simulink model "small_signal_box"  (R2024b)
settings: Solver=VariableStepAuto  StartTime=0.0  StopTime=Tobs  FixedStep=Ts  RelTol=1e-3
values from neighbouring files (symbols this model uses):
  P_finalvalue = 0.486    [main_scan_FD.m]    (also in main_ss_composite.m = 0.05)
  P_initialvalue = storage    (= 0.486)    [main_ss_composite.m]
  P_step = 0.05    [main_ss_composite.m]
  P_step_time = 1.5    [main_scan_FD.m]    (also in main_ss_composite.m = 10)
  Ts = delta_t    (= 1e-05)    [main_scan_FD.m]
  V_finalvalue = 0.99    [main_ss_composite.m]
  V_step_time = 100    [main_scan_FD.m]    (also in main_ss_composite.m = 10)
undefined symbols (not defined in the file or in its folder): C_dc, C_filt, I_charge, ig_d_s, ig_q_s, iL_d_s, iL_q_s, ki_inner_d_pu, ki_inner_q_pu, ki_outer_P_pu, ki_outer_V_pu, ki_pll, kp_inner_d_pu, kp_inner_q_pu, kp_outer_P_pu, kp_outer_V_pu, kp_pll, L, L_base, L_grid, L_vsc, omega_b, P_base, R_grid, R_vsc, t_charge, V_base, V_dc, vdc_mes, vpoc_d_s, vpoc_q_s, vvsc_d_s, vvsc_q_s
libraries: spsabctodq0Lib x8, spsControlledVoltageSourceLib x6, slpidlib x5, spsThreePhaseSeriesRLCBranchLib x3, spsControlledCurrentSourceLib x2, eeGeneralControl x2, spsdq0toabcLib x2, spsThreePhaseVIMeasurementLib x2, spsGroundLib x1, spsLeadLagFilterLib x1, spsParallelRLCBranchLib x1, cstblocks x1
settings Model: SimulationMode=accelerator  Creator=osro  LastModifiedBy=nicolae.darii
settings SolverCC: AlgebraicLoopSolver=TrustRegion
settings DataIOCC: SaveFinalState=on
settings DebuggingCC: UnconnectedInputMsg=warning  UnconnectedOutputMsg=warning  UnconnectedLineMsg=warning
settings ModelReferenceCC: EnableRefExpFcnMdlSchedulingChecks=on
settings RTWCC: GPUComputeCapability=3.5

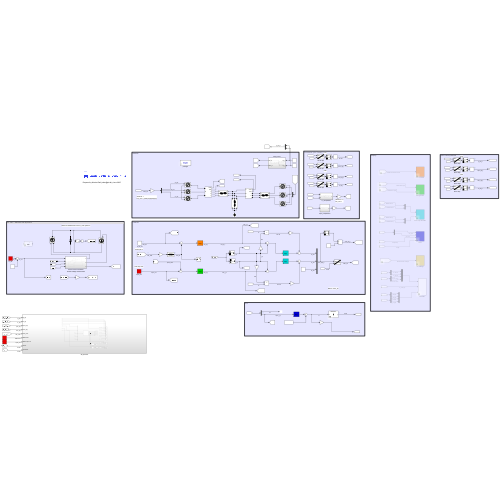
[thumbnail: Simulink's stored preview of the top-level diagram]
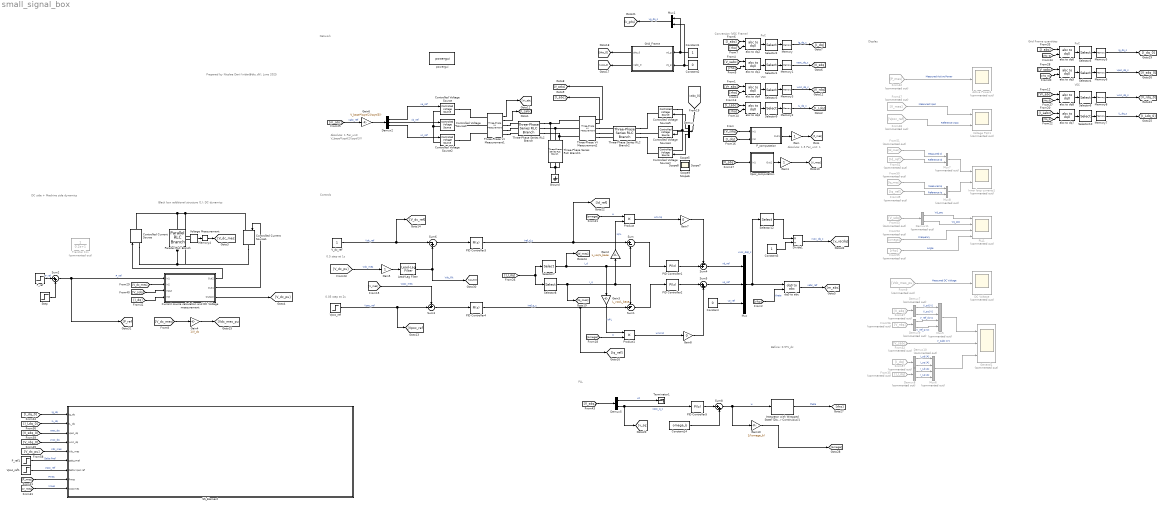
== system small_signal_box ==
  note: Before: 0.5*V_dc
  note: PLL
  note: 0.05 step at 2s
  note: 0.5 step at 1s
  note: Absolute: 1.5
      | Per_unit: 1
  note: Absolute: 1
      | Per_unit: V_base*(sqrt(2)/sqrt(3))
  note: Conversion (VSC Frame)
  note: Controls
  note: Network
  note: VSC
  note: PoC
  note: Prepared by Nicolae Darii (nidar@dtu.dk), June 2025
  note: DC side + Machine side dynamics
  note: Black box additional structure (1): DC dynamics
  note: Display
  note: VSC
  note: Grid Frame quantities
  note: PoC
  Active Power1 : Scope  Commented=on
  Constant : Constant  Value=0
  Constant1 : Constant
  Constant14 : Constant  Value=omega_b
  Constant2 : Constant  Value=0
  Constant3 : Constant
  Controlled Current Source : spsControlledCurrentSourceLib/Controlled Current Source  Initialize=on  Source_Type=AC  Amplitude=0  Phase=0  Frequency=0  Measurements=None
  Controlled Current Source1 : spsControlledCurrentSourceLib/Controlled Current Source  Initialize=on  Source_Type=AC  Amplitude=0  Phase=0  Frequency=0  Measurements=None
  Controlled Voltage Source{,1..5} (6 alike) : spsControlledVoltageSourceLib/Controlled Voltage Source  Initialize=on  Source_Type=AC  Amplitude=0  Phase=0  Frequency=0  Measurements=None
  Current source calculation and DC Voltage measurement : Subsystem
  DC Voltage : Scope  Commented=on
  Demux : Demux  Outputs=3
  Demux{7..11} (5 alike) : Demux  Commented=on  Outputs=2
  Demux2 : Demux  Outputs=3
  Demux5 : Demux  Outputs=2
  Divide1 : Product  Inputs=*/
  From32 : From  Commented=on  GotoTag=V_sabc
  From35 : From  Commented=on  GotoTag=I_Ldq
  From37 : From  Commented=on  GotoTag=V_sdq
  From42 : From  Commented=on  GotoTag=P_mes
  From47 : From  Commented=on  GotoTag=V_mes
  From48 : From  Commented=on  GotoTag=Vpoc_ref
  From49 : From  Commented=on  GotoTag=Iq_ref
  From50 : From  Commented=on  GotoTag=Iq_mes
  From51 : From  Commented=on  GotoTag=Id_mes
  From52 : From  Commented=on  GotoTag=Id_ref
  From53 : From  Commented=on  GotoTag=V_sdq
  From54 : From  Commented=on  GotoTag=omega
  From55 : From  Commented=on  GotoTag=rho
  From56 : From  Commented=on  GotoTag=V_rdq
  From57 : From  Commented=on  GotoTag=I_dq
  From9 : From  Commented=on  GotoTag=Vdc_mes_pu
  Gain : Gain
  Gain1 : Gain
  Gain10 : Gain  Gain=1/(omega_b)
  Gain2 : Gain  Gain=L_vsc/L_base
  Gain3 : Gain  Gain=L_vsc/L_base
  Gain4 : Gain  Gain=1/V_dc
  Gain5 : Gain
  Gain6 : Gain  Gain=V_base*(sqrt(2)/sqrt(3))
  Gain7 : Gain  Gain=0
  Gain8 : Gain  Gain=0
  General1 : Scope  Commented=on  NumInputPorts=3
  Grid_Frame : Subsystem
  Ground : spsGroundLib/Ground  LConnTagsString=a
  Inner loop currents1 : Scope  Commented=on  NumInputPorts=2
  Integrator with Wrapped State (Discrete or Continuous)1 : eeGeneralControl/Integrator with Wrapped State (Discrete or Continuous)  LabelModeActiveChoice=Discrete  WrappedStateUpperValue=2*pi  WrappedStateLowerValue=0  x0=0  Ts=-1
  Lead-Lag Filter : spsLeadLagFilterLib/Lead-Lag Filter  T1=T1  T2=T2  Vdc_Init=1  Ts=Ts
      settings: LibrarySourceBlock=|
      | sps_lib/Control/Filters/Lead-Lag
      | Filter
  Memory{,1..3,5..8} (8 alike) : Memory  InitialCondition=[0 0]  InheritSampleTime=on  LinearizeMemory=on  LinearizeAsDelay=on
  Memory4 : Memory
  Mux : Mux  Inputs=3
  Mux1 : Mux  Inputs=2
  Mux5 : Mux  Commented=on
  Mux6 : Mux  Commented=on
  Mux7 : Mux  Commented=on  Inputs=2
  Mux8 : Mux  Commented=on  Inputs=2
  PID Controller1 : slpidlib/PID Controller  Controller=PI  Form=Parallel  TimeDomain=Discrete-time  UseExternalTs=off  SampleTime=Ts  IntegratorMethod=Forward Euler  FilterMethod=Forward Euler  ControllerParametersSource=internal  P=kp_inner_d_pu  I=ki_inner_d_pu  UseKiTs=off  D=0  UseExternalDerivativeSource=off  N=100  UseFilter=on  TunerSelectOption=Transfer Function Based (PID Tuner App)  InitialConditionSource=internal  InitialConditionForIntegrator=0  InitialConditionForFilter=0  DifferentiatorICPrevScaledInput=0  ExternalReset=none  TrackingMode=off  Kt=1  LimitOutput=off  SatLimitsSource=internal  UpperSaturationLimit=inf  LowerSaturationLimit=-inf  LinearizeAsGain=on  AntiWindupMode=none  Kb=1  LimitIntegrator=off  UpperIntegratorSaturationLimit=inf  LowerIntegratorSaturationLimit=-inf  POutMin=[]  POutMax=[]  IOutMin=[]  IOutMax=[]  DOutMin=[]  DOutMax=[]  NOutMin=[]  NOutMax=[]  SumOutMin=[]  SumOutMax=[]  SaturationOutMin=[]  SaturationOutMax=[]  PParamMin=[]  PParamMax=[]  IParamMin=[]  IParamMax=[]  DParamMin=[]  DParamMax=[]  NParamMin=[]  NParamMax=[]  KbParamMin=[]  KbParamMax=[]  KtParamMin=[]  KtParamMax=[]  KbOutMin=[]  KbOutMax=[]  KtOutMin=[]  KtOutMax=[]  IntegratorOutMin=[]  IntegratorOutMax=[]  FilterOutMin=[]  FilterOutMax=[]  SumI1OutMin=[]  SumI1OutMax=[]  SumI2OutMin=[]  SumI2OutMax=[]  SumI3OutMin=[]  SumI3OutMax=[]  SumI4OutMin=[]  SumI4OutMax=[]  SumDOutMin=[]  SumDOutMax=[]  DifferentiatorOutMin=[]  DifferentiatorOutMax=[]  FilterDiffOutCoefMin=[]  FilterDiffOutCoefMax=[]  ReciprocalOutMin=[]  ReciprocalOutMax=[]  SumDenOutMin=[]  SumDenOutMax=[]  SumNumOutMin=[]  SumNumOutMax=[]  DivideOutMin=[]  DivideOutMax=[]  UdiffTsProdOutMin=[]  UdiffTsProdOutMax=[]  NTsProdOutMin=[]  NTsProdOutMax=[]  UintegralTsProdOutMin=[]  UintegralTsProdOutMax=[]  UngainTsProdOutMin=[]  UngainTsProdOutMax=[]  ClampingZeroOutDataTypeStr=Inherit: Inherit via back propagation  ClampingZeroOutMin=[]  ClampingZeroOutMax=[]  FilterDenConstantOutDataTypeStr=Inherit: Inherit via back propagation  FilterDenConstantOutMin=[]  FilterDenConstantOutMax=[]  PCopyOutDataTypeStr=Inherit: Inherit via back propagation  PCopyOutMin=[]  PCopyOutMax=[]  NCopyOutDataTypeStr=Inherit: Inherit via back propagation  NCopyOutMin=[]  NCopyOutMax=[]  IntegratorContinuousStateAttributes=''  IntegratorStateIdentifier="\"Cd\""  IntegratorStateMustResolveToSignalObject=off  IntegratorRTWStateStorageClass=Auto  FilterContinuousStateAttributes=''  FilterStateMustResolveToSignalObject=off  FilterRTWStateStorageClass=Auto  ParallelPVariant=InternalParameters  IdealPVariant=Disabled  IVariant=InternalParameters  DVariant=Disabled  IntegratorVariant=Discrete  SatVariant=Disabled  AWVariant=Passthrough  PCopyVariant=Disabled  TRVariant=Disabled  FdbkBlocksVariant=Forward  IdealPFdbkVariant=Disabled  SatFdbkVariant=Disabled  DerivativeFilterVariant=Disabled  NVariant=Disabled  NCopyVariant=Disabled_SignalSpec  FilterICVariant=Disabled  IntegratorICVariant=InternalICs  ExternalResetVariant=Disabled  TRSumVariant=Passthrough  SumFdbkVariant=Disabled  SumVariant=Sum_PI  TsampFilterVariant=InternalTs  TsampNgainVariant=Passthrough  TsampIntegralVariant=Disabled_SignalSpec  ExternalSaturationOutDataTypeStr=Inherit: Same as second input  DerivativeSourceVariant=Disabled  PreIntVariant=InternalPreInt
  PID Controller2 : slpidlib/PID Controller  Controller=PI  Form=Parallel  TimeDomain=Discrete-time  UseExternalTs=off  SampleTime=Ts  IntegratorMethod=Forward Euler  FilterMethod=Forward Euler  ControllerParametersSource=internal  P=kp_inner_q_pu  I=ki_inner_q_pu  UseKiTs=off  D=0  UseExternalDerivativeSource=off  N=100  UseFilter=on  TunerSelectOption=Transfer Function Based (PID Tuner App)  InitialConditionSource=internal  InitialConditionForIntegrator=0  InitialConditionForFilter=0  DifferentiatorICPrevScaledInput=0  ExternalReset=none  TrackingMode=off  Kt=1  LimitOutput=off  SatLimitsSource=internal  UpperSaturationLimit=inf  LowerSaturationLimit=-inf  LinearizeAsGain=on  AntiWindupMode=none  Kb=1  LimitIntegrator=off  UpperIntegratorSaturationLimit=inf  LowerIntegratorSaturationLimit=-inf  POutMin=[]  POutMax=[]  IOutMin=[]  IOutMax=[]  DOutMin=[]  DOutMax=[]  NOutMin=[]  NOutMax=[]  SumOutMin=[]  SumOutMax=[]  SaturationOutMin=[]  SaturationOutMax=[]  PParamMin=[]  PParamMax=[]  IParamMin=[]  IParamMax=[]  DParamMin=[]  DParamMax=[]  NParamMin=[]  NParamMax=[]  KbParamMin=[]  KbParamMax=[]  KtParamMin=[]  KtParamMax=[]  KbOutMin=[]  KbOutMax=[]  KtOutMin=[]  KtOutMax=[]  IntegratorOutMin=[]  IntegratorOutMax=[]  FilterOutMin=[]  FilterOutMax=[]  SumI1OutMin=[]  SumI1OutMax=[]  SumI2OutMin=[]  SumI2OutMax=[]  SumI3OutMin=[]  SumI3OutMax=[]  SumI4OutMin=[]  SumI4OutMax=[]  SumDOutMin=[]  SumDOutMax=[]  DifferentiatorOutMin=[]  DifferentiatorOutMax=[]  FilterDiffOutCoefMin=[]  FilterDiffOutCoefMax=[]  ReciprocalOutMin=[]  ReciprocalOutMax=[]  SumDenOutMin=[]  SumDenOutMax=[]  SumNumOutMin=[]  SumNumOutMax=[]  DivideOutMin=[]  DivideOutMax=[]  UdiffTsProdOutMin=[]  UdiffTsProdOutMax=[]  NTsProdOutMin=[]  NTsProdOutMax=[]  UintegralTsProdOutMin=[]  UintegralTsProdOutMax=[]  UngainTsProdOutMin=[]  UngainTsProdOutMax=[]  ClampingZeroOutDataTypeStr=Inherit: Inherit via back propagation  ClampingZeroOutMin=[]  ClampingZeroOutMax=[]  FilterDenConstantOutDataTypeStr=Inherit: Inherit via back propagation  FilterDenConstantOutMin=[]  FilterDenConstantOutMax=[]  PCopyOutDataTypeStr=Inherit: Inherit via back propagation  PCopyOutMin=[]  PCopyOutMax=[]  NCopyOutDataTypeStr=Inherit: Inherit via back propagation  NCopyOutMin=[]  NCopyOutMax=[]  IntegratorContinuousStateAttributes=''  IntegratorStateIdentifier="\"Cq\""  IntegratorStateMustResolveToSignalObject=off  IntegratorRTWStateStorageClass=Auto  FilterContinuousStateAttributes=''  FilterStateMustResolveToSignalObject=off  FilterRTWStateStorageClass=Auto  ParallelPVariant=InternalParameters  IdealPVariant=Disabled  IVariant=InternalParameters  DVariant=Disabled  IntegratorVariant=Discrete  SatVariant=Disabled  AWVariant=Passthrough  PCopyVariant=Disabled  TRVariant=Disabled  FdbkBlocksVariant=Forward  IdealPFdbkVariant=Disabled  SatFdbkVariant=Disabled  DerivativeFilterVariant=Disabled  NVariant=Disabled  NCopyVariant=Disabled_SignalSpec  FilterICVariant=Disabled  IntegratorICVariant=InternalICs  ExternalResetVariant=Disabled  TRSumVariant=Passthrough  SumFdbkVariant=Disabled  SumVariant=Sum_PI  TsampFilterVariant=InternalTs  TsampNgainVariant=Passthrough  TsampIntegralVariant=Disabled_SignalSpec  ExternalSaturationOutDataTypeStr=Inherit: Same as second input  DerivativeSourceVariant=Disabled  PreIntVariant=InternalPreInt
  PID Controller3 : slpidlib/PID Controller  Controller=PI  Form=Parallel  TimeDomain=Discrete-time  UseExternalTs=off  SampleTime=Ts  IntegratorMethod=Forward Euler  FilterMethod=Forward Euler  ControllerParametersSource=internal  P=kp_outer_P_pu  I=ki_outer_P_pu  UseKiTs=off  D=0  UseExternalDerivativeSource=off  N=100  UseFilter=on  TunerSelectOption=Transfer Function Based (PID Tuner App)  InitialConditionSource=internal  InitialConditionForIntegrator=0  InitialConditionForFilter=0  DifferentiatorICPrevScaledInput=0  ExternalReset=none  TrackingMode=off  Kt=1  LimitOutput=off  SatLimitsSource=internal  UpperSaturationLimit=inf  LowerSaturationLimit=-inf  LinearizeAsGain=on  AntiWindupMode=none  Kb=1  LimitIntegrator=off  UpperIntegratorSaturationLimit=inf  LowerIntegratorSaturationLimit=-inf  POutMin=[]  POutMax=[]  IOutMin=[]  IOutMax=[]  DOutMin=[]  DOutMax=[]  NOutMin=[]  NOutMax=[]  SumOutMin=[]  SumOutMax=[]  SaturationOutMin=[]  SaturationOutMax=[]  PParamMin=[]  PParamMax=[]  IParamMin=[]  IParamMax=[]  DParamMin=[]  DParamMax=[]  NParamMin=[]  NParamMax=[]  KbParamMin=[]  KbParamMax=[]  KtParamMin=[]  KtParamMax=[]  KbOutMin=[]  KbOutMax=[]  KtOutMin=[]  KtOutMax=[]  IntegratorOutMin=[]  IntegratorOutMax=[]  FilterOutMin=[]  FilterOutMax=[]  SumI1OutMin=[]  SumI1OutMax=[]  SumI2OutMin=[]  SumI2OutMax=[]  SumI3OutMin=[]  SumI3OutMax=[]  SumI4OutMin=[]  SumI4OutMax=[]  SumDOutMin=[]  SumDOutMax=[]  DifferentiatorOutMin=[]  DifferentiatorOutMax=[]  FilterDiffOutCoefMin=[]  FilterDiffOutCoefMax=[]  ReciprocalOutMin=[]  ReciprocalOutMax=[]  SumDenOutMin=[]  SumDenOutMax=[]  SumNumOutMin=[]  SumNumOutMax=[]  DivideOutMin=[]  DivideOutMax=[]  UdiffTsProdOutMin=[]  UdiffTsProdOutMax=[]  NTsProdOutMin=[]  NTsProdOutMax=[]  UintegralTsProdOutMin=[]  UintegralTsProdOutMax=[]  UngainTsProdOutMin=[]  UngainTsProdOutMax=[]  ClampingZeroOutDataTypeStr=Inherit: Inherit via back propagation  ClampingZeroOutMin=[]  ClampingZeroOutMax=[]  FilterDenConstantOutDataTypeStr=Inherit: Inherit via back propagation  FilterDenConstantOutMin=[]  FilterDenConstantOutMax=[]  PCopyOutDataTypeStr=Inherit: Inherit via back propagation  PCopyOutMin=[]  PCopyOutMax=[]  NCopyOutDataTypeStr=Inherit: Inherit via back propagation  NCopyOutMin=[]  NCopyOutMax=[]  IntegratorContinuousStateAttributes=''  IntegratorStateIdentifier="\"WP\""  IntegratorStateMustResolveToSignalObject=off  IntegratorRTWStateStorageClass=Auto  FilterContinuousStateAttributes=''  FilterStateMustResolveToSignalObject=off  FilterRTWStateStorageClass=Auto  ParallelPVariant=InternalParameters  IdealPVariant=Disabled  IVariant=InternalParameters  DVariant=Disabled  IntegratorVariant=Discrete  SatVariant=Disabled  AWVariant=Passthrough  PCopyVariant=Disabled  TRVariant=Disabled  FdbkBlocksVariant=Forward  IdealPFdbkVariant=Disabled  SatFdbkVariant=Disabled  DerivativeFilterVariant=Disabled  NVariant=Disabled  NCopyVariant=Disabled_SignalSpec  FilterICVariant=Disabled  IntegratorICVariant=InternalICs  ExternalResetVariant=Disabled  TRSumVariant=Passthrough  SumFdbkVariant=Disabled  SumVariant=Sum_PI  TsampFilterVariant=InternalTs  TsampNgainVariant=Passthrough  TsampIntegralVariant=Disabled_SignalSpec  ExternalSaturationOutDataTypeStr=Inherit: Same as second input  DerivativeSourceVariant=Disabled  PreIntVariant=InternalPreInt
  PID Controller4 : slpidlib/PID Controller  Controller=PI  Form=Parallel  TimeDomain=Discrete-time  UseExternalTs=off  SampleTime=Ts  IntegratorMethod=Forward Euler  FilterMethod=Forward Euler  ControllerParametersSource=internal  P=abs(kp_outer_V_pu)  I=abs(ki_outer_V_pu)  UseKiTs=off  D=0  UseExternalDerivativeSource=off  N=100  UseFilter=on  TunerSelectOption=Transfer Function Based (PID Tuner App)  InitialConditionSource=internal  InitialConditionForIntegrator=0  InitialConditionForFilter=0  DifferentiatorICPrevScaledInput=0  ExternalReset=none  TrackingMode=off  Kt=1  LimitOutput=off  SatLimitsSource=internal  UpperSaturationLimit=inf  LowerSaturationLimit=-inf  LinearizeAsGain=on  AntiWindupMode=none  Kb=1  LimitIntegrator=off  UpperIntegratorSaturationLimit=inf  LowerIntegratorSaturationLimit=-inf  POutMin=[]  POutMax=[]  IOutMin=[]  IOutMax=[]  DOutMin=[]  DOutMax=[]  NOutMin=[]  NOutMax=[]  SumOutMin=[]  SumOutMax=[]  SaturationOutMin=[]  SaturationOutMax=[]  PParamMin=[]  PParamMax=[]  IParamMin=[]  IParamMax=[]  DParamMin=[]  DParamMax=[]  NParamMin=[]  NParamMax=[]  KbParamMin=[]  KbParamMax=[]  KtParamMin=[]  KtParamMax=[]  KbOutMin=[]  KbOutMax=[]  KtOutMin=[]  KtOutMax=[]  IntegratorOutMin=[]  IntegratorOutMax=[]  FilterOutMin=[]  FilterOutMax=[]  SumI1OutMin=[]  SumI1OutMax=[]  SumI2OutMin=[]  SumI2OutMax=[]  SumI3OutMin=[]  SumI3OutMax=[]  SumI4OutMin=[]  SumI4OutMax=[]  SumDOutMin=[]  SumDOutMax=[]  DifferentiatorOutMin=[]  DifferentiatorOutMax=[]  FilterDiffOutCoefMin=[]  FilterDiffOutCoefMax=[]  ReciprocalOutMin=[]  ReciprocalOutMax=[]  SumDenOutMin=[]  SumDenOutMax=[]  SumNumOutMin=[]  SumNumOutMax=[]  DivideOutMin=[]  DivideOutMax=[]  UdiffTsProdOutMin=[]  UdiffTsProdOutMax=[]  NTsProdOutMin=[]  NTsProdOutMax=[]  UintegralTsProdOutMin=[]  UintegralTsProdOutMax=[]  UngainTsProdOutMin=[]  UngainTsProdOutMax=[]  ClampingZeroOutDataTypeStr=Inherit: Inherit via back propagation  ClampingZeroOutMin=[]  ClampingZeroOutMax=[]  FilterDenConstantOutDataTypeStr=Inherit: Inherit via back propagation  FilterDenConstantOutMin=[]  FilterDenConstantOutMax=[]  PCopyOutDataTypeStr=Inherit: Inherit via back propagation  PCopyOutMin=[]  PCopyOutMax=[]  NCopyOutDataTypeStr=Inherit: Inherit via back propagation  NCopyOutMin=[]  NCopyOutMax=[]  IntegratorContinuousStateAttributes=''  IntegratorStateIdentifier="\"Flux_PoC\""  IntegratorStateMustResolveToSignalObject=off  IntegratorRTWStateStorageClass=Auto  FilterContinuousStateAttributes=''  FilterStateMustResolveToSignalObject=off  FilterRTWStateStorageClass=Auto  ParallelPVariant=InternalParameters  IdealPVariant=Disabled  IVariant=InternalParameters  DVariant=Disabled  IntegratorVariant=Discrete  SatVariant=Disabled  AWVariant=Passthrough  PCopyVariant=Disabled  TRVariant=Disabled  FdbkBlocksVariant=Forward  IdealPFdbkVariant=Disabled  SatFdbkVariant=Disabled  DerivativeFilterVariant=Disabled  NVariant=Disabled  NCopyVariant=Disabled_SignalSpec  FilterICVariant=Disabled  IntegratorICVariant=InternalICs  ExternalResetVariant=Disabled  TRSumVariant=Passthrough  SumFdbkVariant=Disabled  SumVariant=Sum_PI  TsampFilterVariant=InternalTs  TsampNgainVariant=Passthrough  TsampIntegralVariant=Disabled_SignalSpec  ExternalSaturationOutDataTypeStr=Inherit: Same as second input  DerivativeSourceVariant=Disabled  PreIntVariant=InternalPreInt
  PID Controller5 : slpidlib/PID Controller  Controller=PI  Form=Parallel  TimeDomain=Discrete-time  UseExternalTs=off  SampleTime=Ts  IntegratorMethod=Forward Euler  FilterMethod=Forward Euler  ControllerParametersSource=internal  P=kp_pll  I=ki_pll  UseKiTs=off  D=0  UseExternalDerivativeSource=off  N=100  UseFilter=on  TunerSelectOption=Transfer Function Based (PID Tuner App)  InitialConditionSource=internal  InitialConditionForIntegrator=0  InitialConditionForFilter=0  DifferentiatorICPrevScaledInput=0  ExternalReset=none  TrackingMode=off  Kt=1  LimitOutput=off  SatLimitsSource=internal  UpperSaturationLimit=inf  LowerSaturationLimit=-inf  LinearizeAsGain=on  AntiWindupMode=none  Kb=1  LimitIntegrator=off  UpperIntegratorSaturationLimit=inf  LowerIntegratorSaturationLimit=-inf  POutMin=[]  POutMax=[]  IOutMin=[]  IOutMax=[]  DOutMin=[]  DOutMax=[]  NOutMin=[]  NOutMax=[]  SumOutMin=[]  SumOutMax=[]  SaturationOutMin=[]  SaturationOutMax=[]  PParamMin=[]  PParamMax=[]  IParamMin=[]  IParamMax=[]  DParamMin=[]  DParamMax=[]  NParamMin=[]  NParamMax=[]  KbParamMin=[]  KbParamMax=[]  KtParamMin=[]  KtParamMax=[]  KbOutMin=[]  KbOutMax=[]  KtOutMin=[]  KtOutMax=[]  IntegratorOutMin=[]  IntegratorOutMax=[]  FilterOutMin=[]  FilterOutMax=[]  SumI1OutMin=[]  SumI1OutMax=[]  SumI2OutMin=[]  SumI2OutMax=[]  SumI3OutMin=[]  SumI3OutMax=[]  SumI4OutMin=[]  SumI4OutMax=[]  SumDOutMin=[]  SumDOutMax=[]  DifferentiatorOutMin=[]  DifferentiatorOutMax=[]  FilterDiffOutCoefMin=[]  FilterDiffOutCoefMax=[]  ReciprocalOutMin=[]  ReciprocalOutMax=[]  SumDenOutMin=[]  SumDenOutMax=[]  SumNumOutMin=[]  SumNumOutMax=[]  DivideOutMin=[]  DivideOutMax=[]  UdiffTsProdOutMin=[]  UdiffTsProdOutMax=[]  NTsProdOutMin=[]  NTsProdOutMax=[]  UintegralTsProdOutMin=[]  UintegralTsProdOutMax=[]  UngainTsProdOutMin=[]  UngainTsProdOutMax=[]  ClampingZeroOutDataTypeStr=Inherit: Inherit via back propagation  ClampingZeroOutMin=[]  ClampingZeroOutMax=[]  FilterDenConstantOutDataTypeStr=Inherit: Inherit via back propagation  FilterDenConstantOutMin=[]  FilterDenConstantOutMax=[]  PCopyOutDataTypeStr=Inherit: Inherit via back propagation  PCopyOutMin=[]  PCopyOutMax=[]  NCopyOutDataTypeStr=Inherit: Inherit via back propagation  NCopyOutMin=[]  NCopyOutMax=[]  IntegratorContinuousStateAttributes=''  IntegratorStateIdentifier="\"Flux_PLL\""  IntegratorStateMustResolveToSignalObject=off  IntegratorRTWStateStorageClass=Auto  FilterContinuousStateAttributes=''  FilterStateMustResolveToSignalObject=off  FilterRTWStateStorageClass=Auto  ParallelPVariant=InternalParameters  IdealPVariant=Disabled  IVariant=InternalParameters  DVariant=Disabled  IntegratorVariant=Discrete  SatVariant=Disabled  AWVariant=Passthrough  PCopyVariant=Disabled  TRVariant=Disabled  FdbkBlocksVariant=Forward  IdealPFdbkVariant=Disabled  SatFdbkVariant=Disabled  DerivativeFilterVariant=Disabled  NVariant=Disabled  NCopyVariant=Disabled_SignalSpec  FilterICVariant=Disabled  IntegratorICVariant=InternalICs  ExternalResetVariant=Disabled  TRSumVariant=Passthrough  SumFdbkVariant=Disabled  SumVariant=Sum_PI  TsampFilterVariant=InternalTs  TsampNgainVariant=Passthrough  TsampIntegralVariant=Disabled_SignalSpec  ExternalSaturationOutDataTypeStr=Inherit: Same as second input  DerivativeSourceVariant=Disabled  PreIntVariant=InternalPreInt
  PLL1 : Scope  Commented=on  NumInputPorts=4
  P_computation : Subsystem
  P_ref : Step  Time=P_step_time  After=P_finalvalue  SampleTime=0
  P_ref1 : Step  Time=P_step_time  After=P_step  SampleTime=0
  Parallel RLC Branch : spsParallelRLCBranchLib/Parallel RLC Branch  LConnTagsString=a  RConnTagsString=__new0  BranchType=C  Resistance=1  Inductance=1e-3  SetiL0=off  InitialCurrent=0  Capacitance=C_dc  Setx0=on  InitialVoltage=0  Measurements=None
  Product : Product
  Product1 : Product
  SS_Element : Subsystem
  Selector{1..6,9..10,12} (9 alike) : Selector  InputPortWidth=3  IndexOptions=Index vector (dialog)  Indices=[1 2]  OutputSizes=1
  Selector7 : Selector  InputPortWidth=2  IndexOptions=Index vector (dialog)  Indices=[1]  OutputSizes=1
  Selector8 : Selector  InputPortWidth=2  IndexOptions=Index vector (dialog)  Indices=[2]  OutputSizes=1
  Step : Step  Time=0.5  After=P_initialvalue  SampleTime=0
  Sum : Sum  Inputs=|+-
  Sum1 : Sum  Inputs=-+|
  Sum2 : Sum  Inputs=|++
  Sum3 : Sum  Inputs=+-|
  Sum4 : Sum  Inputs=-+|
  Sum5 : Sum  Inputs=|++
  Sum6 : Sum  Inputs=|-+
  Sum8 : Sum  Inputs=|++
  Terminator1 : Terminator
  Three-Phase Series RLC Branch : spsThreePhaseSeriesRLCBranchLib/Three-Phase Series RLC Branch  LConnTagsString=A|B|C  RConnTagsString=A|B|C  BranchType=RL  Resistance=R_vsc  Inductance=L_vsc  Capacitance=1e-6  Measurements=None
  Three-Phase Series RLC Branch1 : spsThreePhaseSeriesRLCBranchLib/Three-Phase Series RLC Branch  LConnTagsString=A|B|C  RConnTagsString=A|B|C  BranchType=RC  Resistance=0  Inductance=L  Capacitance=C_filt  Measurements=None
  Three-Phase Series RLC Branch2 : spsThreePhaseSeriesRLCBranchLib/Three-Phase Series RLC Branch  LConnTagsString=A|B|C  RConnTagsString=A|B|C  BranchType=RL  Resistance=R_grid  Inductance=L_grid  Capacitance=1e-6  Measurements=None
  Three-Phase V-I Measurement1 : spsThreePhaseVIMeasurementLib/Three-Phase V-I Measurement  VoltageMeasurement=phase-to-ground  SetLabelV=off  LabelV=Vabc  Vpu=on  VpuLL=off  CurrentMeasurement=yes  SetLabelI=off  LabelI=Iabc  Ipu=on  Pbase=P_base  Vbase=V_base  OutputType=Complex  PhasorSimulation=off  PSBequivalent=0
  Three-Phase V-I Measurement2 : spsThreePhaseVIMeasurementLib/Three-Phase V-I Measurement  VoltageMeasurement=phase-to-ground  SetLabelV=off  LabelV=Vabc  Vpu=on  VpuLL=off  CurrentMeasurement=yes  SetLabelI=off  LabelI=Iabc  Ipu=on  Pbase=P_base  Vbase=V_base  OutputType=Complex  PhasorSimulation=off  PSBequivalent=0
  Transfer Fcn : TransferFcn  Commented=on  Denominator=[0.2 1]
  V_dc_ref : Constant
  Voltage Measurement : spsVoltageMeasurementLib/Voltage Measurement  PhasorSimulation=off  OutputType=Complex  PSBequivalent=0
  Voltage PoC1 : Scope  Commented=on  NumInputPorts=2
  Vpoc_computation : Subsystem
  Vpoc_ref : Step  Time=V_step_time  Before=1  After=V_finalvalue  SampleTime=0
  Vpoc_ref1 : Step  Time=V_step_time  After=V_finalvalue-1  SampleTime=0
  abc to dq{1..8} (8 alike) : spsabctodq0Lib/abc to dq0  Alignment=90 degrees behind phase A axis
  dq0 to abc : spsdq0toabcLib/dq0 to abc  Alignment=90 degrees behind phase A axis
  powergui : sps_lib/powergui  Priority=1  SimulationMode=Discrete  SampleTime=Ts  frequency=60  Iterations=50  frequencyindice=0  Pbase=100e6  ErrMax=1e-4  UnitsV=kV  UnitsW=MW  buscounter=0  FunctionMessages=on  echomessages=off  EnableUseOfTLC=off  CurrentSourceSwitches=off  DisableSnubberDevices=off  DisableRonSwitches=off  DisableVfSwitches=off  DisplayEquations=off  AutomaticDiscreteSolvers=off  SolverType=Tustin/Backward Euler (TBE)  Interpol=off  ExternalGateDelay=off  methode=off  Ts=100  x0status=zero  SPID=on  SwTol=0  HookPort=off  NonlinearTolerance=1e-4  nMaxIteration=100  ContinueOnMaxIteration=off  RestoreLinks=warning  ResistiveCurrentMeasurement=off  Frange=[0:2:500]  Ylog=off  Xlog=on  ShowGrid=off  save=off  variable=ZData  structure=0  ZoomFFT=off  StartTime=0.0  cycles=1  DisplayStyle=1  fundamental=60  FreqAxis=off  MaxFrequency=1000  frequencyindicesteady=1  RmsSteady=1  display=off
  Scope{2,5..9} (6 alike) : Scope
  wires:
  Selector1/1 -> Memory1/1
  abc to dq1/1 -> Selector1/1
  [rho] -> dq0 to abc/2  "theta"
  [V_sabc] -> abc to dq1/1
  [rho] -> abc to dq1/2
  [rho] -> abc to dq2/2
  Selector2/1 -> Memory/1
  [I_abc] -> abc to dq2/1
  abc to dq2/1 -> Selector2/1
  Constant/1 -> Mux/3  "v0_ref"
  Memory/1 -> [I_dq]  "Ig_dq_c"
  Memory1/1 -> [V_sdq]  "vpoc_dq_c"
  Memory2/1 -> [I_Ldq]  "iL_dq_c"
  abc to dq3/1 -> Selector9/1
  [I_Labc] -> abc to dq3/1
  Selector9/1 -> Memory2/1
  [rho] -> abc to dq3/2
  [V_sdq] -> P_computation/1(In1)
  [I_dq] -> P_computation/2(In2)
  P_computation/1(Out1) -> Gain/1
  [V_sdq] -> Vpoc_computation/1(In1)
  Vpoc_computation/1(Out1) -> Gain1/1
  Selector7/1 -> [Id_mes], Sum/2, Gain3/1  "I_d"
  [I_Ldq] -> Selector7/1, Selector8/1
  Selector8/1 -> [Iq_mes], Sum1/1, Gain2/1  "I_q"
  Sum/1 -> PID Controller1/1
  Sum1/1 -> PID Controller2/1
  [rho] -> abc to dq4/2
  Selector3/1 -> Memory3/1
  Memory3/1 -> [V_rdq]  "vvsc_dq_c"
  abc to dq4/1 -> Selector3/1
  [Vr_abc] -> abc to dq4/1
  Sum3/1 -> PID Controller4/1
  [V_mes] -> Sum3/1  "Vpoc_mes"
  Vpoc_ref/1 -> [Vpoc_ref], Sum3/2  "Vpoc_ref"
  dq0 to abc/1 -> [m_abc]  "vabc_ref"
  Gain/1 -> [P_mes]
  Gain1/1 -> [V_mes]
  PID Controller4/1 -> [Iq_ref], Sum1/2  "iref_q_c"
  [omega] -> Product/1  "w"
  Gain2/1 -> Product/2  "Iq*L"
  [omega] -> Product1/2  "w"
  Gain3/1 -> Product1/1  "Id*L"
  PID Controller1/1 -> Sum4/2
  Sum4/1 -> Mux/1  "vd_ref"
  Product/1 -> Gain7/1  "w*L*Iq"
  PID Controller2/1 -> Sum5/1
  Sum5/1 -> Mux/2  "vq_ref"
  Product1/1 -> Gain8/1  "w*L*Id"
  PID Controller3/1 -> [Id_ref], Sum/1  "iref_d_c"
  Demux5/1 -> Terminator1/1  "vd"
  [V_sdq] -> Demux5/1
  Demux5/2 -> [v_sq], PID Controller5/1  "vpoc_q_c"
  Constant14/1 -> Sum8/2
  Sum8/1 -> Gain10/1, Integrator with Wrapped State (Discrete or Continuous)1/1  "w"
  PID Controller5/1 -> Sum8/1
  Integrator with Wrapped State (Discrete or Continuous)1/1 -> [rho]  "theta"
  Mux/1 -> Selector12/1, dq0 to abc/1  "vvsc_dq0_c"
  Gain10/1 -> [omega]
  [V_sdq] -> Current source calculation and DC Voltage measurement/3(Input)
  Voltage Measurement/1 -> Memory4/1
  Current source calculation and DC Voltage measurement/1(Out2) -> Controlled Current Source/1
  [I_dq] -> Current source calculation and DC Voltage measurement/4(In3)
  Current source calculation and DC Voltage measurement/2(Out1) -> Controlled Current Source1/1
  Memory4/1 -> [V_dc_mes]
  Current source calculation and DC Voltage measurement/3(Output) -> [V_dc_pu]
  [V_dc_mes] -> Current source calculation and DC Voltage measurement/2(In2)
  Sum2/1 -> Current source calculation and DC Voltage measurement/1(In1), [P_ref]  "P_ref"
  Sum6/1 -> PID Controller3/1
  V_dc_ref/1 -> [V_dc_ref], Sum6/1  "Vdc_ref"
  Demux9/2 -> Mux5/4  "V_ref_q [V]"
  From9/1 -> DC Voltage/1  "Measured DC Voltage"
  From55/1 -> PLL1/4  "Angle"
  From35/1 -> Demux8/1
  From57/1 -> Demux10/1
  From54/1 -> PLL1/3  "Frequency"
  From47/1 -> Voltage PoC1/1  "Measured Vpoc"
  Demux11/2 -> PLL1/2  "Vq_poc"
  Demux8/2 -> Mux6/4  "I_Lq [A]"
  From50/1 -> Mux8/1  "Measured Iq"
  Demux10/1 -> Mux6/1  "I_sd [A]"
  Mux6/1 -> General1/3
  Demux11/1 -> PLL1/1  "Vd_poc"
  Demux7/2 -> Mux5/2  "V_sq [V]"
  From51/1 -> Mux7/1  "Measured Id"
  From56/1 -> Demux9/1
  Demux8/1 -> Mux6/3  "I_Ld [A]"
  From48/1 -> Voltage PoC1/2  "Reference Vpoc"
  From53/1 -> Demux11/1
  From49/1 -> Mux8/2  "Reference Iq"
  Mux8/1 -> Inner loop currents1/2
  From42/1 -> Active Power1/1  "Measured Active Power"
  Mux5/1 -> General1/1
  From32/1 -> General1/2  "V_sabc [V]"
  Demux10/2 -> Mux6/2  "I_sq [A]"
  Demux7/1 -> Mux5/1  "V_sd [V]"
  Demux9/1 -> Mux5/3  "V_ref_d [V]"
  From52/1 -> Mux7/2  "Reference Id"
  Mux7/1 -> Inner loop currents1/1
  From37/1 -> Demux7/1
  [V_dc_mes] -> Gain4/1
  Gain4/1 -> [Vdc_mes_pu]
  [V_dc_pu] -> Gain5/1  "Vdc_mes"
  Gain5/1 -> Lead-Lag Filter/1
  Lead-Lag Filter/1 -> Sum6/2, [Vdc_filt]  "Vdc_filt"
  Grid_Frame/1(pho_0) -> [rho_0]
  Grid_Frame/2(vabc_0) -> [vabc_0]
  [m_abc] -> Gain6/1  "vabc_ref"
  Demux2/1 -> Controlled Voltage Source/1  "va_ref"
  Demux2/2 -> Controlled Voltage Source1/1  "vb_ref"
  Demux2/3 -> Controlled Voltage Source2/1  "vc_ref"
  Three-Phase V-I Measurement1/1 -> [Vr_abc]
  Three-Phase V-I Measurement1/2 -> [I_Labc]
  Three-Phase V-I Measurement2/1 -> [V_sabc]
  Three-Phase V-I Measurement2/2 -> [I_abc]
  Constant1/1 -> Mux1/1, Grid_Frame/1(vd_g)
  Constant2/1 -> Mux1/2, Grid_Frame/2(vq_g)
  Demux/1 -> Controlled Voltage Source5/1
  Demux/2 -> Controlled Voltage Source4/1
  Demux/3 -> Controlled Voltage Source3/1
  [vabc_0] -> Demux/1
  abc to dq7/1 -> Selector10/1
  Memory5/1 -> [I_dq_0]  "ig_dq_s"
  [Vr_abc] -> abc to dq8/1
  [rho_0] -> abc to dq7/2
  [I_Labc] -> abc to dq7/1
  [I_abc] -> abc to dq6/1
  Selector6/1 -> Memory8/1
  [rho_0] -> abc to dq6/2
  Selector4/1 -> Memory6/1
  abc to dq8/1 -> Selector6/1
  [V_sabc] -> abc to dq5/1
  [rho_0] -> abc to dq5/2
  abc to dq5/1 -> Selector4/1
  Memory8/1 -> [V_rdq_0]  "vvsc_dq_s"
  abc to dq6/1 -> Selector5/1
  Selector5/1 -> Memory5/1
  Memory6/1 -> [V_sdq_0]  "vpoc_dq_s"
  Memory7/1 -> [I_Ldq_0]  "iL_dq_s"
  Selector10/1 -> Memory7/1
  [rho_0] -> abc to dq8/2
  Gain6/1 -> Demux2/1
  Mux1/1 -> [v_gdq]  "vg_dq_s"
  Step/1 -> Sum2/2
  P_ref/1 -> Sum2/1  "P_ref"
  [I_Ldq_0] -> SS_Element/2(iL_dq)  "iL_dq"
  [V_sdq_0] -> SS_Element/3(vpoc_dq)  "vpoc_dq"
  [V_rdq_0] -> SS_Element/4(vvsc_dq)  "vvsc_dq"
  [V_dc_pu] -> SS_Element/5(Vdc_mes)  "Vdc_mes"
  P_ref1/1 -> SS_Element/6(Delta Pref)  "Delta Pref"
  [I_dq_0] -> SS_Element/1(ig_dq)  "ig_dq"
  Vpoc_ref1/1 -> SS_Element/7(Delta Vpoc ref)  "Vpoc_ref"
  Gain7/1 -> Sum4/1
  Gain8/1 -> Sum5/2
  Divide1/1 -> [v_vscdq]  "vvsc_dq_c"
  [P_mes] -> SS_Element/8(Pmes)  "Pmes"
  [V_mes] -> SS_Element/9(Vpocmes)  "Vmes"
  Constant3/1 -> Divide1/2
  Selector12/1 -> Divide1/1
  connections:
  Parallel RLC Branch/RConn1 -- Controlled Current Source/LConn1 -- Controlled Current Source1/RConn1 -- Voltage Measurement/LConn2
  Voltage Measurement/LConn1 -- Controlled Current Source/RConn1 -- Parallel RLC Branch/LConn1 -- Controlled Current Source1/LConn1
  Controlled Voltage Source5/LConn1 -- Controlled Voltage Source4/LConn1 -- Controlled Voltage Source3/LConn1
  Controlled Voltage Source1/LConn1 -- Controlled Voltage Source2/LConn1 -- Controlled Voltage Source/LConn1
  Controlled Voltage Source/RConn1 -- Three-Phase V-I Measurement1/LConn1
  Controlled Voltage Source1/RConn1 -- Three-Phase V-I Measurement1/LConn2
  Controlled Voltage Source2/RConn1 -- Three-Phase V-I Measurement1/LConn3
  Three-Phase V-I Measurement1/RConn1 -- Three-Phase Series RLC Branch/LConn1
  Three-Phase V-I Measurement1/RConn2 -- Three-Phase Series RLC Branch/LConn2
  Three-Phase V-I Measurement1/RConn3 -- Three-Phase Series RLC Branch/LConn3
  Three-Phase Series RLC Branch/RConn1 -- Three-Phase V-I Measurement2/LConn1 -- Three-Phase Series RLC Branch1/LConn1
  Three-Phase Series RLC Branch/RConn2 -- Three-Phase Series RLC Branch1/LConn2 -- Three-Phase V-I Measurement2/LConn2
  Three-Phase Series RLC Branch/RConn3 -- Three-Phase Series RLC Branch1/LConn3 -- Three-Phase V-I Measurement2/LConn3
  Three-Phase Series RLC Branch1/RConn1 -- Ground/LConn1 -- Three-Phase Series RLC Branch1/RConn3 -- Three-Phase Series RLC Branch1/RConn2
  Three-Phase V-I Measurement2/RConn1 -- Three-Phase Series RLC Branch2/LConn1
  Three-Phase V-I Measurement2/RConn2 -- Three-Phase Series RLC Branch2/LConn2
  Three-Phase V-I Measurement2/RConn3 -- Three-Phase Series RLC Branch2/LConn3
  Three-Phase Series RLC Branch2/RConn1 -- Controlled Voltage Source5/RConn1
  Three-Phase Series RLC Branch2/RConn2 -- Controlled Voltage Source4/RConn1
  Three-Phase Series RLC Branch2/RConn3 -- Controlled Voltage Source3/RConn1

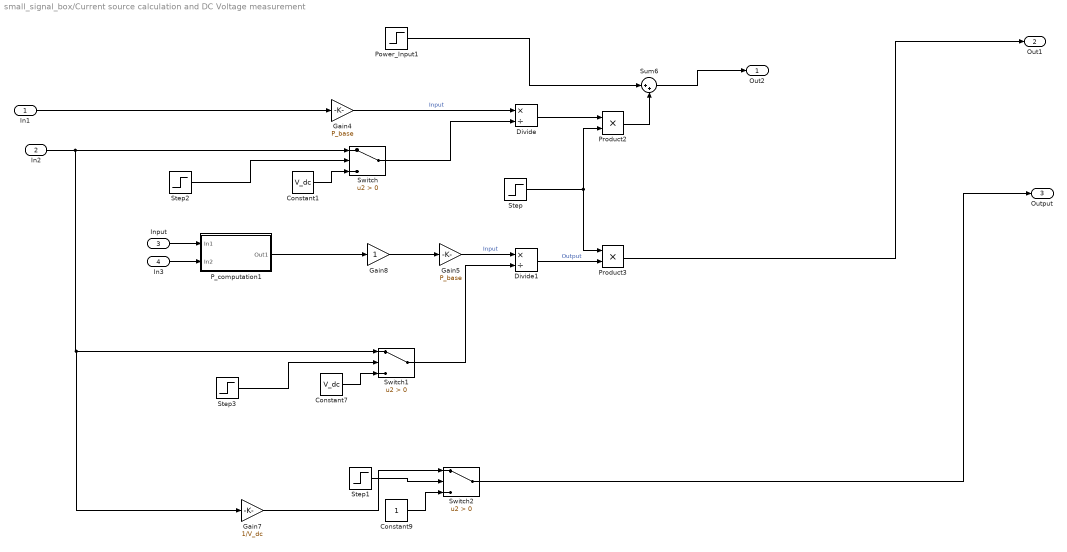
== system small_signal_box/Current source calculation and DC Voltage measurement ==
  In1 : Inport
  In2 : Inport  Port=2
  Input : Inport  Port=3
  In3 : Inport  Port=4
  Constant1 : Constant  Value=V_dc
  Constant7 : Constant  Value=V_dc
  Constant9 : Constant
  Divide : Product  Inputs=*/
  Divide1 : Product  Inputs=*/
  Gain4 : Gain  Gain=P_base
  Gain5 : Gain  Gain=P_base
  Gain7 : Gain  Gain=1/V_dc
  Gain8 : Gain
  P_computation1 : Subsystem
  Power_Input1 : Step  Time=t_charge  Before=I_charge  After=0  SampleTime=0
  Product2 : Product
  Product3 : Product
  Step : Step  Time=t_charge + 0.1  SampleTime=0
  Step1 : Step  Time=0.6  SampleTime=0
  Step2 : Step  Time=0.1  SampleTime=0
  Step3 : Step  Time=0.1  SampleTime=0
  Sum6 : Sum  Inputs=|++
  Switch : Switch  Criteria=u2 > Threshold  SaturateOnIntegerOverflow=off  InputSameDT=off
  Switch1 : Switch  Criteria=u2 > Threshold  SaturateOnIntegerOverflow=off  InputSameDT=off
  Switch2 : Switch  Criteria=u2 > Threshold  SaturateOnIntegerOverflow=off  InputSameDT=off
  Out2 : Outport
  Out1 : Outport  Port=2
  Output : Outport  Port=3
  wires:
  Step3/1 -> Switch1/2
  In1/1 -> Gain4/1
  Constant1/1 -> Switch/3
  Product3/1 -> Out1/1
  Step/1 -> Product3/1, Product2/2
  Divide/1 -> Product2/1
  Gain8/1 -> Gain5/1
  Constant7/1 -> Switch1/3
  Divide1/1 -> Product3/2  "Output"
  Product2/1 -> Sum6/2
  Gain5/1 -> Divide1/1  "Input"
  Power_Input1/1 -> Sum6/1
  Step2/1 -> Switch/2
  P_computation1/1(Out1) -> Gain8/1
  Switch/1 -> Divide/2
  Gain4/1 -> Divide/1  "Input"
  Switch1/1 -> Divide1/2
  Sum6/1 -> Out2/1
  Input/1 -> P_computation1/1(In1)
  In3/1 -> P_computation1/2(In2)
  Step1/1 -> Switch2/2
  Switch2/1 -> Output/1
  Gain7/1 -> Switch2/1
  In2/1 -> Gain7/1, Switch1/1, Switch/1
  Constant9/1 -> Switch2/3

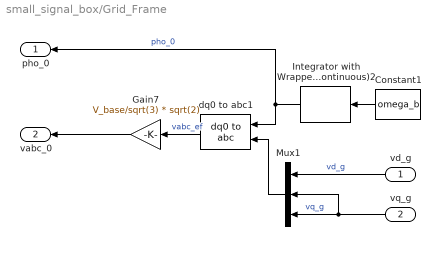
== system small_signal_box/Grid_Frame ==
  vd_g : Inport
  vq_g : Inport  Port=2
  Constant1 : Constant  Value=omega_b
  Gain7 : Gain  Gain=V_base/sqrt(3) * sqrt(2)
  Integrator with Wrapped State (Discrete or Continuous)2 : eeGeneralControl/Integrator with Wrapped State (Discrete or Continuous)  LabelModeActiveChoice=Discrete  WrappedStateUpperValue=2*pi  WrappedStateLowerValue=0  x0=0  Ts=-1
  Mux1 : Mux  Inputs=3
  dq0 to abc1 : spsdq0toabcLib/dq0 to abc  Alignment=90 degrees behind phase A axis
  pho_0 : Outport
  vabc_0 : Outport  Port=2
  wires:
  Constant1/1 -> Integrator with Wrapped State (Discrete or Continuous)2/1
  Integrator with Wrapped State (Discrete or Continuous)2/1 -> pho_0/1, dq0 to abc1/2  "pho_0"
  Mux1/1 -> dq0 to abc1/1
  dq0 to abc1/1 -> Gain7/1  "vabc_ef"
  Gain7/1 -> vabc_0/1
  vd_g/1 -> Mux1/1  "vd_g"
  vq_g/1 -> Mux1/3, Mux1/2  "vq_g"

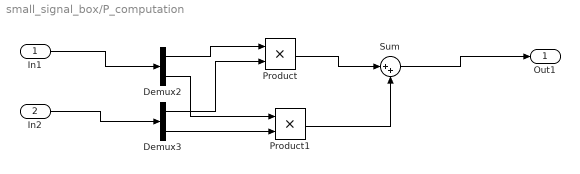
== system small_signal_box/P_computation ==
  In1 : Inport
  In2 : Inport  Port=2
  Demux2 : Demux  Outputs=2
  Demux3 : Demux  Outputs=2
  Product : Product
  Product1 : Product
  Sum : Sum  Inputs=|++
  Out1 : Outport
  wires:
  In1/1 -> Demux2/1
  In2/1 -> Demux3/1
  Demux2/1 -> Product/1
  Demux3/1 -> Product/2
  Demux2/2 -> Product1/1
  Demux3/2 -> Product1/2
  Product/1 -> Sum/1
  Product1/1 -> Sum/2
  Sum/1 -> Out1/1

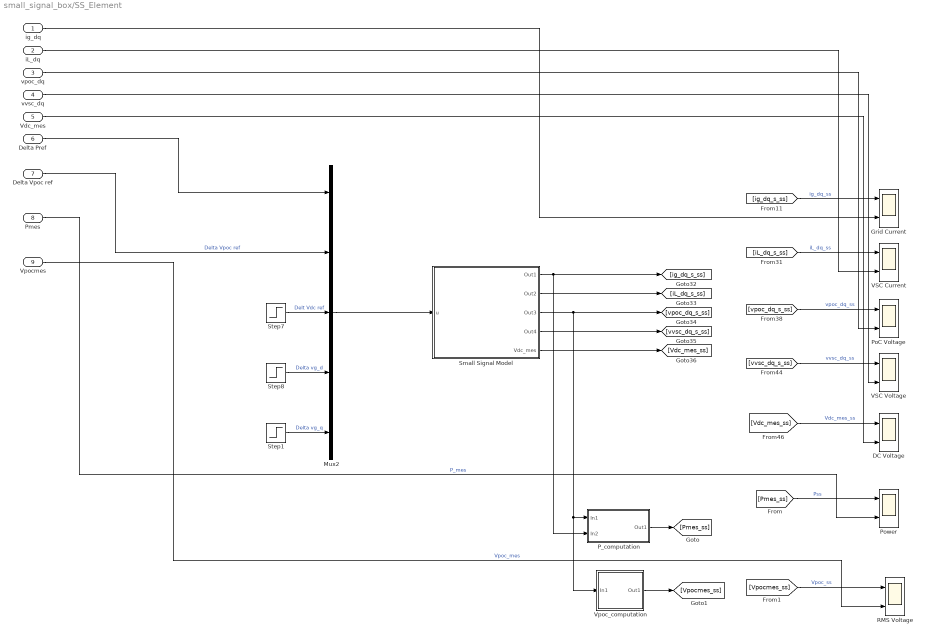
== system small_signal_box/SS_Element ==
  ig_dq : Inport
  iL_dq : Inport  Port=2
  vpoc_dq : Inport  Port=3
  vvsc_dq : Inport  Port=4
  Vdc_mes : Inport  Port=5
  Delta Pref : Inport  Port=6
  Delta Vpoc ref : Inport  Port=7
  Pmes : Inport  Port=8
  Vpocmes : Inport  Port=9
  DC Voltage : Scope  NumInputPorts=2
  Grid Current : Scope  NumInputPorts=2
  Mux2 : Mux  Inputs=5
  P_computation : Subsystem
  PoC Voltage : Scope  NumInputPorts=2
  Power : Scope  NumInputPorts=2
  RMS Voltage : Scope  NumInputPorts=2
  Small Signal Model : Subsystem
  Step1 : Step  Time=100  After=0.5  SampleTime=0
  Step7 : Step  Time=100  After=0.5  SampleTime=0
  Step8 : Step  Time=100  After=-0.05  SampleTime=0
  VSC Current : Scope  NumInputPorts=2
  VSC Voltage : Scope  NumInputPorts=2
  Vpoc_computation : Subsystem
  wires:
  Mux2/1 -> Small Signal Model/1(u)
  Small Signal Model/4(Out4) -> [vvsc_dq_s_ss]
  vpoc_dq/1 -> PoC Voltage/2
  Small Signal Model/5(Vdc_mes) -> [Vdc_mes_ss]
  [vpoc_dq_s_ss] -> PoC Voltage/1  "vpoc_dq_ss"
  Delta Vpoc ref/1 -> Mux2/2  "Delta Vpoc ref"
  Step7/1 -> Mux2/3  "Delt Vdc ref"
  Small Signal Model/1(Out1) -> [ig_dq_s_ss], P_computation/2(In2)
  Step8/1 -> Mux2/4  "Delta vg_d"
  Small Signal Model/3(Out3) -> [vpoc_dq_s_ss], Vpoc_computation/1(In1), P_computation/1(In1)
  Step1/1 -> Mux2/5  "Delta vg_q"
  [vvsc_dq_s_ss] -> VSC Voltage/1  "vvsc_dq_ss"
  vvsc_dq/1 -> VSC Voltage/2
  [iL_dq_s_ss] -> VSC Current/1  "iL_dq_ss"
  Small Signal Model/2(Out2) -> [iL_dq_s_ss]
  [ig_dq_s_ss] -> Grid Current/1  "ig_dq_ss"
  [Vdc_mes_ss] -> DC Voltage/1  "Vdc_mes_ss"
  iL_dq/1 -> VSC Current/2
  ig_dq/1 -> Grid Current/2
  Vdc_mes/1 -> DC Voltage/2
  Delta Pref/1 -> Mux2/1
  P_computation/1(Out1) -> [Pmes_ss]
  [Pmes_ss] -> Power/1  "Pss"
  Pmes/1 -> Power/2  "P_mes"
  Vpoc_computation/1(Out1) -> [Vpocmes_ss]
  [Vpocmes_ss] -> RMS Voltage/1  "Vpoc_ss"
  Vpocmes/1 -> RMS Voltage/2  "Vpoc_mes"

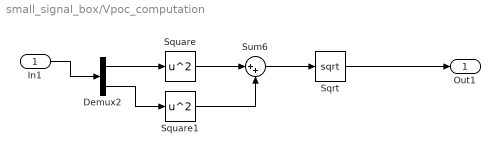
== system small_signal_box/Vpoc_computation ==
  In1 : Inport
  Demux2 : Demux  Outputs=2
  Sqrt : Sqrt
  Square : Math  Operator=square
  Square1 : Math  Operator=square
  Sum6 : Sum  Inputs=|++
  Out1 : Outport
  wires:
  Sqrt/1 -> Out1/1
  Sum6/1 -> Sqrt/1
  Demux2/1 -> Square/1
  Square1/1 -> Sum6/2
  In1/1 -> Demux2/1
  Square/1 -> Sum6/1
  Demux2/2 -> Square1/1

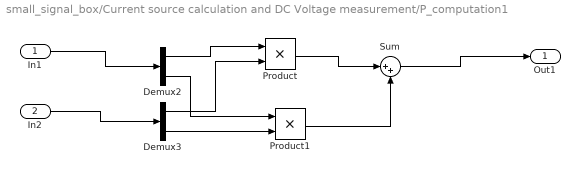
== system small_signal_box/Current source calculation and DC Voltage measurement/P_computation1 ==
  In1 : Inport
  In2 : Inport  Port=2
  Demux2 : Demux  Outputs=2
  Demux3 : Demux  Outputs=2
  Product : Product
  Product1 : Product
  Sum : Sum  Inputs=|++
  Out1 : Outport
  wires:
  In1/1 -> Demux2/1
  In2/1 -> Demux3/1
  Demux2/1 -> Product/1
  Demux3/1 -> Product/2
  Demux2/2 -> Product1/1
  Demux3/2 -> Product1/2
  Product/1 -> Sum/1
  Product1/1 -> Sum/2
  Sum/1 -> Out1/1

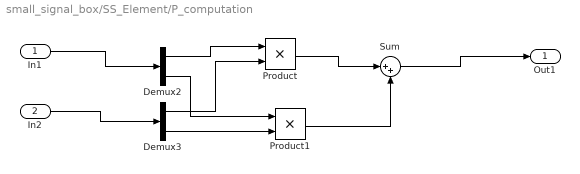
== system small_signal_box/SS_Element/P_computation ==
  In1 : Inport
  In2 : Inport  Port=2
  Demux2 : Demux  Outputs=2
  Demux3 : Demux  Outputs=2
  Product : Product
  Product1 : Product
  Sum : Sum  Inputs=|++
  Out1 : Outport
  wires:
  In1/1 -> Demux2/1
  In2/1 -> Demux3/1
  Demux2/1 -> Product/1
  Demux3/1 -> Product/2
  Demux2/2 -> Product1/1
  Demux3/2 -> Product1/2
  Product/1 -> Sum/1
  Product1/1 -> Sum/2
  Sum/1 -> Out1/1

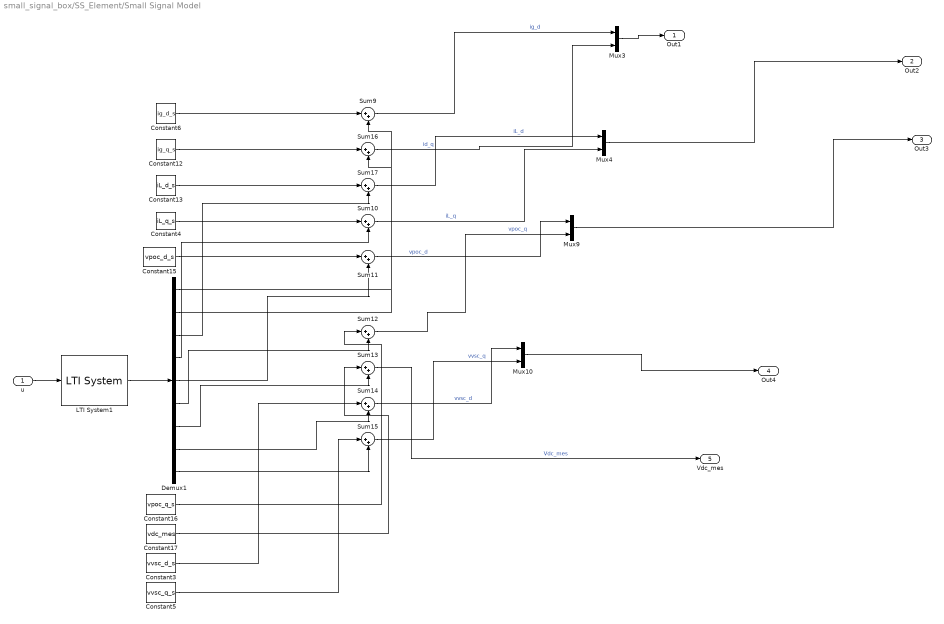
== system small_signal_box/SS_Element/Small Signal Model ==
  u : Inport
  Constant12 : Constant  Value=ig_q_s
  Constant13 : Constant  Value=iL_d_s
  Constant15 : Constant  Value=vpoc_d_s
  Constant16 : Constant  Value=vpoc_q_s
  Constant17 : Constant  Value=vdc_mes
  Constant3 : Constant  Value=vvsc_d_s
  Constant4 : Constant  Value=iL_q_s
  Constant5 : Constant  Value=vvsc_q_s
  Constant6 : Constant  Value=ig_d_s
  Demux1 : Demux  Outputs=9
  LTI System1 : cstblocks/LTI System  sys=ss_system  IC=[]  PadeOrder=0
  Mux{3..4,9..10} (4 alike) : Mux  Inputs=2
  Sum{9..17} (9 alike) : Sum  Inputs=|++
  Out1 : Outport
  Out2 : Outport  Port=2
  Out3 : Outport  Port=3
  Out4 : Outport  Port=4
  Vdc_mes : Outport  Port=5
  wires:
  Demux1/5 -> Sum11/2
  Demux1/4 -> Sum10/2
  Constant12/1 -> Sum16/1
  Mux9/1 -> Out3/1
  Demux1/7 -> Sum13/2
  Sum11/1 -> Mux9/1  "vpoc_d"
  Constant5/1 -> Sum15/1
  Constant17/1 -> Sum13/1
  Sum15/1 -> Mux10/2  "vvsc_q"
  Mux4/1 -> Out2/1
  Demux1/2 -> Sum16/2
  Demux1/3 -> Sum17/2
  Constant13/1 -> Sum17/1
  Demux1/8 -> Sum14/2
  LTI System1/1 -> Demux1/1
  Sum12/1 -> Mux9/2  "vpoc_q"
  Constant3/1 -> Sum14/1
  Sum17/1 -> Mux4/1  "iL_d"
  Demux1/1 -> Sum9/2
  Constant15/1 -> Sum11/1
  Mux3/1 -> Out1/1
  Sum14/1 -> Mux10/1  "vvsc_d"
  Constant6/1 -> Sum9/1
  Constant16/1 -> Sum12/1
  Sum10/1 -> Mux4/2  "iL_q"
  Sum9/1 -> Mux3/1  "ig_d"
  Demux1/9 -> Sum15/2
  Constant4/1 -> Sum10/1
  Mux10/1 -> Out4/1
  Demux1/6 -> Sum12/2
  Sum16/1 -> Mux3/2  "id_q"
  u/1 -> LTI System1/1
  Sum13/1 -> Vdc_mes/1  "Vdc_mes"

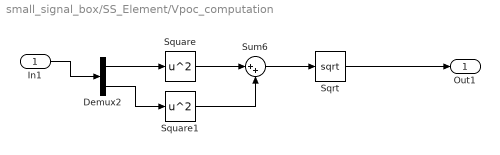
== system small_signal_box/SS_Element/Vpoc_computation ==
  In1 : Inport
  Demux2 : Demux  Outputs=2
  Sqrt : Sqrt
  Square : Math  Operator=square
  Square1 : Math  Operator=square
  Sum6 : Sum  Inputs=|++
  Out1 : Outport
  wires:
  Sqrt/1 -> Out1/1
  Sum6/1 -> Sqrt/1
  Demux2/1 -> Square/1
  Square1/1 -> Sum6/2
  In1/1 -> Demux2/1
  Square/1 -> Sum6/1
  Demux2/2 -> Square1/1
